simulink model "Ex_simpledcmotor_SL"  (R2024b)
settings: Solver=VariableStepAuto  StartTime=0.0  StopTime=10.0  RelTol=1e-3
PreLoadFcn:
  | load("properties.mat");
undefined symbols (not defined in the file): b, J, K, L, R, V
settings Model: Creator=gsasaki  LastModifiedBy=agarcian
settings OptimizationCC: DefaultParameterBehavior=Inlined  UseDivisionForNetSlopeComputation=on  GainParamInheritBuiltInType=on  UseFloatMulNetSlope=on  InlineInvariantSignals=on  PassReuseOutputArgsAs=Individual arguments  ZeroExternalMemoryAtStartup=off  ZeroInternalMemoryAtStartup=off  NoFixptDivByZeroProtection=on  EfficientFloat2IntCast=on  LifeSpan=1  OptimizeBlockOrder=speed  DifferentSizesBufferReuse=on  EfficientTunableParamExpr=on
settings DebuggingCC: ParameterTunabilityLossMsg=error  UnconnectedInputMsg=warning  UnconnectedOutputMsg=warning  UnconnectedLineMsg=warning
settings HardwareCC: ProdLongLongMode=on
settings ModelReferenceCC: EnableRefExpFcnMdlSchedulingChecks=on
settings SFSimCC: MATLABDynamicMemAlloc=off
settings RTWCC: Description=Embedded Coder  SystemTargetFile=ert.tlc  TemplateMakefile=ert_default_tmf  GPUComputeCapability=3.5  DLArmComputeVersion=19.05
settings CodeAppCC: ForceParamTrailComments=on  IgnoreCustomStorageClasses=off  OperatorAnnotations=on  SimulinkDataObjDesc=on  SFDataObjDesc=on  CustomSymbolStrGlobalVar=rt$N$M  CustomSymbolStrType=$N$M  CustomSymbolStrFcn=$N$M$F  CustomSymbolStrMacro=$N$M  InsertBlockDesc=on
settings ERTTargetCC: TargetLangStandard=C99 (ISO)  GenerateSampleERTMain=on  IncludeMdlTerminateFcn=off  CombineSignalStateStructs=on  SupportAbsoluteTime=off  SupportComplex=off  SupportContinuousTime=on  ERTCustomFileTemplate=example_file_process.tlc  ERTFilePackagingFormat=CompactWithDataFile  DynamicArrayContainerType=coder::array

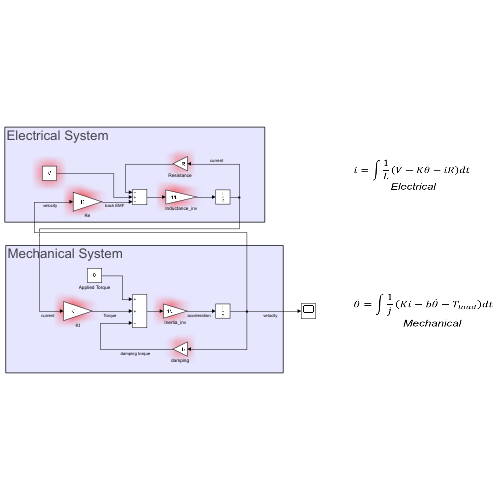
[thumbnail: Simulink's stored preview of the top-level diagram]
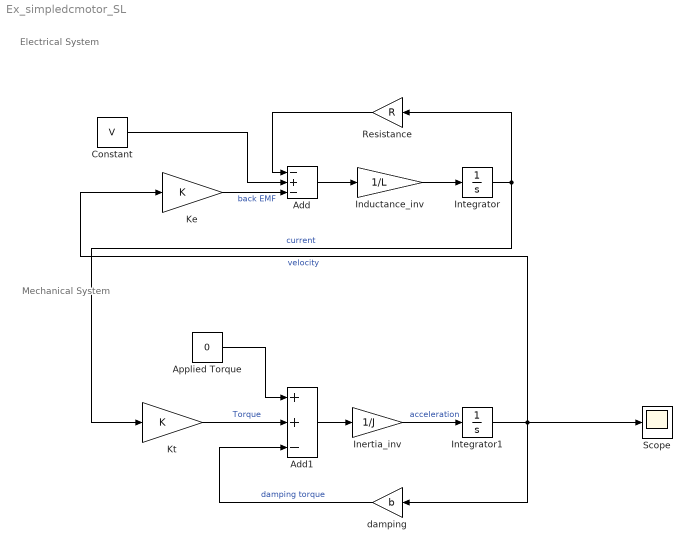
== system Ex_simpledcmotor_SL ==
  note: Mechanical System
  note: Electrical System
  Add : Sum  Inputs=-+-
  Add1 : Sum  Inputs=++-
  Applied Torque : Constant  Value=0
  Constant : Constant  Value=V
  Inductance_inv : Gain  Gain=1/L
  Inertia_inv : Gain  Gain=1/J
  Integrator : Integrator
  Integrator1 : Integrator
  Ke : Gain  Gain=K
  Kt : Gain  Gain=K
  Resistance : Gain  Gain=R
  Scope : Scope
  damping : Gain  Gain=b
  wires:
  Ke/1 -> Add/3  "back EMF"
  Inductance_inv/1 -> Integrator/1
  Add/1 -> Inductance_inv/1
  Integrator/1 -> Kt/1, Resistance/1  "current"
  Resistance/1 -> Add/1
  Kt/1 -> Add1/2  "Torque"
  Add1/1 -> Inertia_inv/1
  Inertia_inv/1 -> Integrator1/1  "acceleration"
  Integrator1/1 -> Scope/1, Ke/1, damping/1  "velocity"
  damping/1 -> Add1/3  "damping torque"
  Applied Torque/1 -> Add1/1
  Constant/1 -> Add/2
